simulink model "RealtimeModel"  (Simulink 7.0)
settings: Solver=FixedStepDiscrete  SolverMode=MultiTasking  StartTime=0.0  StopTime=RunningTime  FixedStep=sample  RelTol=1e-3
values from neighbouring files (symbols this model uses):
  Integrator = InitializeIntegrator(Integrator, Structure)    [RealtimeModel_Setup.m]
  Interpolations = SampleRate/sample    [RealtimeModel_Setup.m]
  sample = 1/1024    (= 0.0009765625)    [RealtimeModel_Setup.m]
  SampleRate = Integrator.Timestep    [RealtimeModel_Setup.m]
undefined symbols (not defined in the file or in its folder): Elements
(part 3 of 3)

== matlab function Generate Element Restoring Forces/Generate Type 3 Element Restoring Force Element 2/Type 3 Element RF ==
  data: TotalRF output inherited; Element input inherited; a1 input inherited; a2 input inherited; pmx input inherited; bmy_init input inherited; Displacement input inherited; NumFreeDOF parameter inherited
% Get Restoring Force Type 3
function TotalRF  = fnc(Element, a1, a2, pmx, bmy_init, Displacement, NumFreeDOF)

persistent initialized;
persistent kody;
persistent bmep;
persistent bmel;
persistent bmtot;
persistent bbmy;
persistent dpr;
persistent bmy;
persistent ftot;
persistent pracn;
persistent pracp;
persistent prtot;
persistent sftot;
persistent Uprev;

%% Input mapping
ksurf = Element(1);
cosa = Element(2);
eal = Element(3);
ek11 = Element(4);
ek11h = Element(5);
ek12 = Element(6);
ek22 = Element(7);
ek22h = Element(8);
fl = Element(9);
pr12 = Element(10);
pr21 = Element(11);
psh = Element(12);
sina = Element(13);
Node1UX = Element(14);
Node1UY = Element(15);
Node1THETA = Element(16);
Node2UX = Element(17);
Node2UY = Element(18);
Node2THETA = Element(19);

if isempty(initialized)
    initialized = 1;
    kody = zeros(2,1);
    bmep = zeros(2,1); 
    bmel = zeros(2,1);
    bmtot = zeros(2,1);
    bbmy = 0;
    dpr = zeros(2,1);
    ftot = zeros(2,1);  
    pracn = zeros(2,1); 
    pracp = zeros(2,1);
    prtot = zeros(2,1);
    sftot = zeros(2,1); 
    Uprev = zeros(6,1);
    bmy = bmy_init;
end

%% Get the displacement Ue (6x1) vector of the element in global coordinates
Ue = zeros(6,1);
dof=zeros(6,1);
dof(1,1)=Node1UX;
dof(2,1)=Node1UY;
dof(3,1)=Node1THETA;
dof(4,1)=Node2UX;
dof(5,1)=Node2UY;
dof(6,1)=Node2THETA;
for i=1:6
    if dof(i,1)<=NumFreeDOF
        Ue(i,1)=Displacement(dof(i,1),1);
    end
end

%% Input of Drain State Determination Type 2 Element
ndof=6;  %the element has 6 dofs
ddise=Ue-Uprev;  %the incremental displacement vector ddise of the element in global coordinates 
Uprev=Ue; %update Uprev of element for use in next state determination call
%% calculate element deformation increments
[dvax,dvr] = ELDFO2(ddise,fl,cosa,sina);
%% UPDATE AXIAL FORCES AND AXIAL ENERGY
dfax=eal*dvax;      
ftot(1,1)=ftot(1,1)-dfax;
ftot(2,1)=ftot(2,1)+dfax;  
%% MOMENTS IN ELASTIC COMPONENT AT BEGINING OF STEP
bmel(1,1)=bmtot(1,1)-bmep(1,1);
bmel(2,1)=bmtot(2,1)-bmep(2,1);
%% LINEAR MOMENT INCREMENTS FOR ELASTO-PLASTIC COMPONENT - SET IN DBM
[dbm] = BMCAO2(dvr,kody,ek11,ek12,ek22,ek22h,ek11h);
%% TRACE NONLINEAR PATH FOR ELASTO-PLASTIC COMPONENT---state determination
facac=0.0;
while (facac<0.999999)
    factor=1.0-facac;
    % PLASTIC HINGE ROTATIONS
    kod=kody(1,1)+kody(2,1)-1.0;
    if(kod>0)
        % hinges at both ends
        dpr(1,1)=dvr(1,1);
        dpr(2,1)=dvr(2,1);
    elseif(kod==0)
        % hinge at one end only
        dpr(1,1)=dvr(1,1)+pr21*dvr(2,1);
        dpr(2,1)=dvr(2,1)+pr12*dvr(1,1);
    else
         %never executed
    end
         
    % CALCULATE WHICH END HAS NEXT EVENT IF YIELDS, SET KFAC=IEND AND BBMY=YIELD VALUE
    % SET EVENT FACTOR IN FACTOR
    kfac=3;
    for iend=1:2
        if (kody(iend,1)==0.0)
            dbmm=dbm(iend,1);
            % elastic, get factor for status change(no hinge at end)
            if (dbmm<0.0)
                dbmo=bmy(iend,2)-bmep(iend,1);
                if(dbmo>=dbmm) 
                    fac=dbmo/dbmm;
                else
                    fac=2.0;
                end 
                if (fac<=factor)
                    factor=fac;
                    bbmy=bmy(iend,2);
                    kfac=iend;
                end
            elseif(dbmm>0.0)
                dbmo=bmy(iend,1)-bmep(iend,1);
                if(dbmo<=dbmm) 
                    fac=dbmo/dbmm;
                else
                    fac=2.0;
                end 
                if (fac<=factor)
                    factor=fac;
                    bbmy=bmy(iend,1);
                    kfac=iend;
                end
            else
            end
        else
            % hinge at this end
            if(bmep(iend,1)*dpr(iend,1)<0.0)
            % unloading (plastic work negative)
                factor=0.0;
                kfac=0.0;
                kody(iend,1)=0.0;
            else
                % continuing to yield (plastic work positive)
            end
        end
    end
    % UPDATE BENDING STATE AND CALCULATE BENDING ENERGY
    % dbm= elastic increment - use if elastic bbmy= yield value - use if yields
    if(kfac~=0)
        for iend=1:2
            if(iend==kfac)
                % new hinge at this end
                bmep(iend,1)=bbmy;
                kody(iend,1)=1;
            elseif(kody(iend,1)==0)
                % this end remains elastic
                dmep=factor*dbm(iend,1);
                bmep(iend,1)=bmep(iend,1)+dmep;
            else
                % this end remains plastic
                dppr=factor*dpr(iend,1);
                prtot(iend,1)=prtot(iend,1)+dppr;
                if (dppr<0.0)
                    pracn(iend,1)=pracn(iend,1)+dppr;
                else
                    pracp(iend,1)=pracp(iend,1)+dppr;
                end
            end
        end
    else
        % unloads - factor=0.
    end
    % CHECK COMPLETION OF CYCLE
    facac=facac+factor;
    if (facac<0.99999)
        % cycle not completed, calculate new moment increments
        [dbm] = BMCAO2(dvr,kody,ek11,ek12,ek22,ek22h,ek11h);
    end
end
%% YIELD MOMENTS FOR NEXT STEP
if(ksurf==1)
    [bmy] = YMOM02(ftot,pmx,a1,a2,bmy);
    % CHECK YIELD SURFACE OVERSHOOT
    for iend=1:2
        if (kody(iend,1)~=0.0)
        % inelastic on old surface
            if (bmep(iend,1)>bmy(iend,1)) 
                % inelastic positive on new surface also
                bmep(iend,1)=bmy(iend,1);
            elseif (bmep(iend,1)<bmy(iend,2))
                % inelastic negative on new surface also
                bmep(iend,1)=bmy(iend,2);
            elseif ((bmep(iend,1)<(bmy(iend,1)*0.98)) && (bmep(iend,1)>(bmy(iend,2)*0.98)))
                % moves inside new surface by > 2% - reset yield code
                kody(iend,1)=0;
            else
            end
        else
            % elastic on old surface
            if (bmep(iend,1)>bmy(iend,1))
                % inelastic positive on new surface
                bmep(iend,1)=bmy(iend,1);
                kody(iend,1)=1;
            elseif (bmep(iend,1)<=bmy(iend,2))
                % inelastic negative on new surface
                bmep(iend,1)=bmy(iend,2);
                kody(iend,1)=1;
            else
            end
        end
    end
end
%% UPDATE TOTAL FORCES
dsf=(bmtot(1,1)+ bmtot(2,1))/fl;
ppsh=psh/(1.0-psh);
dmeli=(ek11*dvr(1,1)+ek12*dvr(2,1))*ppsh+bmel(1,1);
dmelj=(ek12*dvr(1,1)+ ek22*dvr(2,1))*ppsh+bmel(2,1);
bmtot(1,1)=bmep(1,1)+dmeli;
bmtot(2,1)=bmep(2,1)+dmelj;
dsf=dsf-(bmtot(1,1)+bmtot(2,1))/fl;
sftot(1,1)=sftot(1,1)-dsf;
sftot(2,1)=sftot(2,1)+dsf;

RF = ELASO2(ndof,ftot,cosa,sina,sftot,bmtot);

% Form total restoring force vector
TotalRF = zeros(NumFreeDOF, 1);
    
% Get element nodes to assemble in the structure restoring force vector
if Node1UX <= NumFreeDOF
    TotalRF(Node1UX, 1) = RF(1, 1);
end
if Node1UY <= NumFreeDOF
    TotalRF(Node1UY, 1) = RF(2, 1);
end
if Node1THETA <= NumFreeDOF
    TotalRF(Node1THETA, 1) = RF(3, 1);
end
if Node2UX <= NumFreeDOF
    TotalRF(Node2UX, 1) = RF(4, 1);
end
if Node2UY <= NumFreeDOF
    TotalRF(Node2UY, 1) = RF(5, 1);
end
if Node2THETA <= NumFreeDOF
    TotalRF(Node2THETA, 1) = RF(6, 1);
end





%%%%%%% FUNCTIONS %%%%%%%%%
function [bmy] = YMOM02(ftot,pmx,a1,a2,bmy)
facc=-1.0;
for iend = 1 : 2
    % Change sign of axial force and end 1
    fft = ftot(iend,1) * facc;
    facc = 1;
    fac = 1;
    for j = 1 : 2
        fac = -fac;
        yieldcalc = 0;  % flag if the yield moment is calculated inside 
                        % this next for loop
        for i = 1 : 3
            if (fft < pmx(i,j,iend))
                yieldcalc = 1;  % set flag since the condition was met
                % Calculate yield moment (M = a2 + a1P)
                bbmy = a2(i,j,iend) - a1(i,j,iend) * fft;
                if (fac * bbmy > 0) 
                    % Axial force is beyond Pc and Pt
                    bbmy = 0;
                end
                bmy(iend,j) = bbmy;
            end
        end
        % Only calculate yield moment if it wasn't calculated in the above
        % for loop
        if (yieldcalc == 0)
            i = 4;
            % Calculate yield moment (M = a2 + a1P)
            bbmy = a2(i,j,iend) - a1(i,j,iend) * fft;
            if (fac * bbmy > 0) 
                % Axial force is beyond Pc and Pt
                bbmy = 0;
            end
            bmy(iend,j) = bbmy;
        end
    end
end
%c ---------------------------------INTERCHANGE BMY(1,1) AND BMY(1,2) AND
%c ------------------------------AND ALSO CHANGE SIGN OF MOMENTS AT END 1
fac=-bmy(1,1);
bmy(1,1)=-bmy(1,2);
bmy(1,2)=fac;
      
      
      
      
      
function [dbm] = BMCAO2(dvr,kody,ek11,ek12,ek22,ek22h,ek11h)
dbm=zeros(2,1);
% c ------------------SET KYY TO INDICATE TYPE OF ELEMENT STIFFNESS TO USE
      kyy=kody(1,1)+2*kody(2,1)+1;
      if(kyy==1)
%c---no hinge at either end
        dbm(1,1)=ek11*dvr(1,1)+ek12*dvr(2,1);
        dbm(2,1)=ek12*dvr(1,1)+ek22*dvr(2,1);
      elseif(kyy==2)
%c---hinge at end 1
        dbm(1,1)=0.0;
        dbm(2,1)=ek22h*dvr(2,1);
      elseif(kyy==3)
%c---hinge at end 2
        dbm(1,1)=ek11h*dvr(1,1);
        dbm(2,1)=0.0;
      elseif(kyy==4)
%c---hinges at both end
        dbm(1,1)=0.0;
        dbm(2,1)=0.0;
       else
           %never executed
      end
      
      
      
      
      
      
      
      
      
      
   %%
function [relas] = ELASO2(ndof,ftot,cosa,sina,sftot,bmtot)
%%
relas=zeros(ndof,1);
%BASIC RESISTING FORCES
      relas(1,1)=(ftot(1,1)-0)*cosa-(sftot(1,1)-0)*sina;
      relas(2,1)=(ftot(1,1)-0)*sina+(sftot(1,1)-0)*cosa;
      relas(3,1)=bmtot(1,1)-0-0;
      relas(4,1)=(ftot(2,1)-0)*cosa-(sftot(2,1)-0)*sina;
      relas(5,1)=(ftot(2,1)-0)*sina+(sftot(2,1)-0)*cosa;
      relas(6,1)=bmtot(2,1)-0-0;
%%







%%
function [dvax,dvr] = ELDFO2(ddise,f1,cosa, sina) 
%%
dvr=zeros(2,1);
%DEFORMATION INCREMENTS OR DEFORMATION RATES
      dvax=cosa*(ddise(4,1)-ddise(1,1))+sina*(ddise(5,1)-ddise(2,1));
      rot=(sina*(ddise(4,1)-ddise(1,1))+cosa*(ddise(2,1)-ddise(5,1)))/f1;
      dvr(1,1)=ddise(3,1)+rot;
      dvr(2,1)=ddise(6,1)+rot;
%%

== matlab function Generate Element Restoring Forces/Generate Type 3 Element Restoring Force Element 4/Type 3 Element RF ==
  data: TotalRF output inherited; Element input inherited; a1 input inherited; a2 input inherited; pmx input inherited; bmy_init input inherited; Displacement input inherited; NumFreeDOF parameter inherited
% Get Restoring Force Type 3
function TotalRF  = fnc(Element, a1, a2, pmx, bmy_init, Displacement, NumFreeDOF)

persistent initialized;
persistent kody;
persistent bmep;
persistent bmel;
persistent bmtot;
persistent bbmy;
persistent dpr;
persistent bmy;
persistent ftot;
persistent pracn;
persistent pracp;
persistent prtot;
persistent sftot;
persistent Uprev;

%% Input mapping
ksurf = Element(1);
cosa = Element(2);
eal = Element(3);
ek11 = Element(4);
ek11h = Element(5);
ek12 = Element(6);
ek22 = Element(7);
ek22h = Element(8);
fl = Element(9);
pr12 = Element(10);
pr21 = Element(11);
psh = Element(12);
sina = Element(13);
Node1UX = Element(14);
Node1UY = Element(15);
Node1THETA = Element(16);
Node2UX = Element(17);
Node2UY = Element(18);
Node2THETA = Element(19);

if isempty(initialized)
    initialized = 1;
    kody = zeros(2,1);
    bmep = zeros(2,1); 
    bmel = zeros(2,1);
    bmtot = zeros(2,1);
    bbmy = 0;
    dpr = zeros(2,1);
    ftot = zeros(2,1);  
    pracn = zeros(2,1); 
    pracp = zeros(2,1);
    prtot = zeros(2,1);
    sftot = zeros(2,1); 
    Uprev = zeros(6,1);
    bmy = bmy_init;
end

%% Get the displacement Ue (6x1) vector of the element in global coordinates
Ue = zeros(6,1);
dof=zeros(6,1);
dof(1,1)=Node1UX;
dof(2,1)=Node1UY;
dof(3,1)=Node1THETA;
dof(4,1)=Node2UX;
dof(5,1)=Node2UY;
dof(6,1)=Node2THETA;
for i=1:6
    if dof(i,1)<=NumFreeDOF
        Ue(i,1)=Displacement(dof(i,1),1);
    end
end

%% Input of Drain State Determination Type 2 Element
ndof=6;  %the element has 6 dofs
ddise=Ue-Uprev;  %the incremental displacement vector ddise of the element in global coordinates 
Uprev=Ue; %update Uprev of element for use in next state determination call
%% calculate element deformation increments
[dvax,dvr] = ELDFO2(ddise,fl,cosa,sina);
%% UPDATE AXIAL FORCES AND AXIAL ENERGY
dfax=eal*dvax;      
ftot(1,1)=ftot(1,1)-dfax;
ftot(2,1)=ftot(2,1)+dfax;  
%% MOMENTS IN ELASTIC COMPONENT AT BEGINING OF STEP
bmel(1,1)=bmtot(1,1)-bmep(1,1);
bmel(2,1)=bmtot(2,1)-bmep(2,1);
%% LINEAR MOMENT INCREMENTS FOR ELASTO-PLASTIC COMPONENT - SET IN DBM
[dbm] = BMCAO2(dvr,kody,ek11,ek12,ek22,ek22h,ek11h);
%% TRACE NONLINEAR PATH FOR ELASTO-PLASTIC COMPONENT---state determination
facac=0.0;
while (facac<0.999999)
    factor=1.0-facac;
    % PLASTIC HINGE ROTATIONS
    kod=kody(1,1)+kody(2,1)-1.0;
    if(kod>0)
        % hinges at both ends
        dpr(1,1)=dvr(1,1);
        dpr(2,1)=dvr(2,1);
    elseif(kod==0)
        % hinge at one end only
        dpr(1,1)=dvr(1,1)+pr21*dvr(2,1);
        dpr(2,1)=dvr(2,1)+pr12*dvr(1,1);
    else
         %never executed
    end
         
    % CALCULATE WHICH END HAS NEXT EVENT IF YIELDS, SET KFAC=IEND AND BBMY=YIELD VALUE
    % SET EVENT FACTOR IN FACTOR
    kfac=3;
    for iend=1:2
        if (kody(iend,1)==0.0)
            dbmm=dbm(iend,1);
            % elastic, get factor for status change(no hinge at end)
            if (dbmm<0.0)
                dbmo=bmy(iend,2)-bmep(iend,1);
                if(dbmo>=dbmm) 
                    fac=dbmo/dbmm;
                else
                    fac=2.0;
                end 
                if (fac<=factor)
                    factor=fac;
                    bbmy=bmy(iend,2);
                    kfac=iend;
                end
            elseif(dbmm>0.0)
                dbmo=bmy(iend,1)-bmep(iend,1);
                if(dbmo<=dbmm) 
                    fac=dbmo/dbmm;
                else
                    fac=2.0;
                end 
                if (fac<=factor)
                    factor=fac;
                    bbmy=bmy(iend,1);
                    kfac=iend;
                end
            else
            end
        else
            % hinge at this end
            if(bmep(iend,1)*dpr(iend,1)<0.0)
            % unloading (plastic work negative)
                factor=0.0;
                kfac=0.0;
                kody(iend,1)=0.0;
            else
                % continuing to yield (plastic work positive)
            end
        end
    end
    % UPDATE BENDING STATE AND CALCULATE BENDING ENERGY
    % dbm= elastic increment - use if elastic bbmy= yield value - use if yields
    if(kfac~=0)
        for iend=1:2
            if(iend==kfac)
                % new hinge at this end
                bmep(iend,1)=bbmy;
                kody(iend,1)=1;
            elseif(kody(iend,1)==0)
                % this end remains elastic
                dmep=factor*dbm(iend,1);
                bmep(iend,1)=bmep(iend,1)+dmep;
            else
                % this end remains plastic
                dppr=factor*dpr(iend,1);
                prtot(iend,1)=prtot(iend,1)+dppr;
                if (dppr<0.0)
                    pracn(iend,1)=pracn(iend,1)+dppr;
                else
                    pracp(iend,1)=pracp(iend,1)+dppr;
                end
            end
        end
    else
        % unloads - factor=0.
    end
    % CHECK COMPLETION OF CYCLE
    facac=facac+factor;
    if (facac<0.99999)
        % cycle not completed, calculate new moment increments
        [dbm] = BMCAO2(dvr,kody,ek11,ek12,ek22,ek22h,ek11h);
    end
end
%% YIELD MOMENTS FOR NEXT STEP
if(ksurf==1)
    [bmy] = YMOM02(ftot,pmx,a1,a2,bmy);
    % CHECK YIELD SURFACE OVERSHOOT
    for iend=1:2
        if (kody(iend,1)~=0.0)
        % inelastic on old surface
            if (bmep(iend,1)>bmy(iend,1)) 
                % inelastic positive on new surface also
                bmep(iend,1)=bmy(iend,1);
            elseif (bmep(iend,1)<bmy(iend,2))
                % inelastic negative on new surface also
                bmep(iend,1)=bmy(iend,2);
            elseif ((bmep(iend,1)<(bmy(iend,1)*0.98)) && (bmep(iend,1)>(bmy(iend,2)*0.98)))
                % moves inside new surface by > 2% - reset yield code
                kody(iend,1)=0;
            else
            end
        else
            % elastic on old surface
            if (bmep(iend,1)>bmy(iend,1))
                % inelastic positive on new surface
                bmep(iend,1)=bmy(iend,1);
                kody(iend,1)=1;
            elseif (bmep(iend,1)<=bmy(iend,2))
                % inelastic negative on new surface
                bmep(iend,1)=bmy(iend,2);
                kody(iend,1)=1;
            else
            end
        end
    end
end
%% UPDATE TOTAL FORCES
dsf=(bmtot(1,1)+ bmtot(2,1))/fl;
ppsh=psh/(1.0-psh);
dmeli=(ek11*dvr(1,1)+ek12*dvr(2,1))*ppsh+bmel(1,1);
dmelj=(ek12*dvr(1,1)+ ek22*dvr(2,1))*ppsh+bmel(2,1);
bmtot(1,1)=bmep(1,1)+dmeli;
bmtot(2,1)=bmep(2,1)+dmelj;
dsf=dsf-(bmtot(1,1)+bmtot(2,1))/fl;
sftot(1,1)=sftot(1,1)-dsf;
sftot(2,1)=sftot(2,1)+dsf;

RF = ELASO2(ndof,ftot,cosa,sina,sftot,bmtot);

% Form total restoring force vector
TotalRF = zeros(NumFreeDOF, 1);
    
% Get element nodes to assemble in the structure restoring force vector
if Node1UX <= NumFreeDOF
    TotalRF(Node1UX, 1) = RF(1, 1);
end
if Node1UY <= NumFreeDOF
    TotalRF(Node1UY, 1) = RF(2, 1);
end
if Node1THETA <= NumFreeDOF
    TotalRF(Node1THETA, 1) = RF(3, 1);
end
if Node2UX <= NumFreeDOF
    TotalRF(Node2UX, 1) = RF(4, 1);
end
if Node2UY <= NumFreeDOF
    TotalRF(Node2UY, 1) = RF(5, 1);
end
if Node2THETA <= NumFreeDOF
    TotalRF(Node2THETA, 1) = RF(6, 1);
end





%%%%%%% FUNCTIONS %%%%%%%%%
function [bmy] = YMOM02(ftot,pmx,a1,a2,bmy)
facc=-1.0;
for iend = 1 : 2
    % Change sign of axial force and end 1
    fft = ftot(iend,1) * facc;
    facc = 1;
    fac = 1;
    for j = 1 : 2
        fac = -fac;
        yieldcalc = 0;  % flag if the yield moment is calculated inside 
                        % this next for loop
        for i = 1 : 3
            if (fft < pmx(i,j,iend))
                yieldcalc = 1;  % set flag since the condition was met
                % Calculate yield moment (M = a2 + a1P)
                bbmy = a2(i,j,iend) - a1(i,j,iend) * fft;
                if (fac * bbmy > 0) 
                    % Axial force is beyond Pc and Pt
                    bbmy = 0;
                end
                bmy(iend,j) = bbmy;
            end
        end
        % Only calculate yield moment if it wasn't calculated in the above
        % for loop
        if (yieldcalc == 0)
            i = 4;
            % Calculate yield moment (M = a2 + a1P)
            bbmy = a2(i,j,iend) - a1(i,j,iend) * fft;
            if (fac * bbmy > 0) 
                % Axial force is beyond Pc and Pt
                bbmy = 0;
            end
            bmy(iend,j) = bbmy;
        end
    end
end
%c ---------------------------------INTERCHANGE BMY(1,1) AND BMY(1,2) AND
%c ------------------------------AND ALSO CHANGE SIGN OF MOMENTS AT END 1
fac=-bmy(1,1);
bmy(1,1)=-bmy(1,2);
bmy(1,2)=fac;
      
      
      
      
      
function [dbm] = BMCAO2(dvr,kody,ek11,ek12,ek22,ek22h,ek11h)
dbm=zeros(2,1);
% c ------------------SET KYY TO INDICATE TYPE OF ELEMENT STIFFNESS TO USE
      kyy=kody(1,1)+2*kody(2,1)+1;
      if(kyy==1)
%c---no hinge at either end
        dbm(1,1)=ek11*dvr(1,1)+ek12*dvr(2,1);
        dbm(2,1)=ek12*dvr(1,1)+ek22*dvr(2,1);
      elseif(kyy==2)
%c---hinge at end 1
        dbm(1,1)=0.0;
        dbm(2,1)=ek22h*dvr(2,1);
      elseif(kyy==3)
%c---hinge at end 2
        dbm(1,1)=ek11h*dvr(1,1);
        dbm(2,1)=0.0;
      elseif(kyy==4)
%c---hinges at both end
        dbm(1,1)=0.0;
        dbm(2,1)=0.0;
       else
           %never executed
      end
      
      
      
      
      
      
      
      
      
      
   %%
function [relas] = ELASO2(ndof,ftot,cosa,sina,sftot,bmtot)
%%
relas=zeros(ndof,1);
%BASIC RESISTING FORCES
      relas(1,1)=(ftot(1,1)-0)*cosa-(sftot(1,1)-0)*sina;
      relas(2,1)=(ftot(1,1)-0)*sina+(sftot(1,1)-0)*cosa;
      relas(3,1)=bmtot(1,1)-0-0;
      relas(4,1)=(ftot(2,1)-0)*cosa-(sftot(2,1)-0)*sina;
      relas(5,1)=(ftot(2,1)-0)*sina+(sftot(2,1)-0)*cosa;
      relas(6,1)=bmtot(2,1)-0-0;
%%







%%
function [dvax,dvr] = ELDFO2(ddise,f1,cosa, sina) 
%%
dvr=zeros(2,1);
%DEFORMATION INCREMENTS OR DEFORMATION RATES
      dvax=cosa*(ddise(4,1)-ddise(1,1))+sina*(ddise(5,1)-ddise(2,1));
      rot=(sina*(ddise(4,1)-ddise(1,1))+cosa*(ddise(2,1)-ddise(5,1)))/f1;
      dvr(1,1)=ddise(3,1)+rot;
      dvr(2,1)=ddise(6,1)+rot;
%%

== matlab function Generate Element Restoring Forces/Generate Type 3 Element Restoring Force Element 5/Type 3 Element RF ==
  data: TotalRF output inherited; Element input inherited; a1 input inherited; a2 input inherited; pmx input inherited; bmy_init input inherited; Displacement input inherited; NumFreeDOF parameter inherited
% Get Restoring Force Type 3
function TotalRF  = fnc(Element, a1, a2, pmx, bmy_init, Displacement, NumFreeDOF)

persistent initialized;
persistent kody;
persistent bmep;
persistent bmel;
persistent bmtot;
persistent bbmy;
persistent dpr;
persistent bmy;
persistent ftot;
persistent pracn;
persistent pracp;
persistent prtot;
persistent sftot;
persistent Uprev;

%% Input mapping
ksurf = Element(1);
cosa = Element(2);
eal = Element(3);
ek11 = Element(4);
ek11h = Element(5);
ek12 = Element(6);
ek22 = Element(7);
ek22h = Element(8);
fl = Element(9);
pr12 = Element(10);
pr21 = Element(11);
psh = Element(12);
sina = Element(13);
Node1UX = Element(14);
Node1UY = Element(15);
Node1THETA = Element(16);
Node2UX = Element(17);
Node2UY = Element(18);
Node2THETA = Element(19);

if isempty(initialized)
    initialized = 1;
    kody = zeros(2,1);
    bmep = zeros(2,1); 
    bmel = zeros(2,1);
    bmtot = zeros(2,1);
    bbmy = 0;
    dpr = zeros(2,1);
    ftot = zeros(2,1);  
    pracn = zeros(2,1); 
    pracp = zeros(2,1);
    prtot = zeros(2,1);
    sftot = zeros(2,1); 
    Uprev = zeros(6,1);
    bmy = bmy_init;
end

%% Get the displacement Ue (6x1) vector of the element in global coordinates
Ue = zeros(6,1);
dof=zeros(6,1);
dof(1,1)=Node1UX;
dof(2,1)=Node1UY;
dof(3,1)=Node1THETA;
dof(4,1)=Node2UX;
dof(5,1)=Node2UY;
dof(6,1)=Node2THETA;
for i=1:6
    if dof(i,1)<=NumFreeDOF
        Ue(i,1)=Displacement(dof(i,1),1);
    end
end

%% Input of Drain State Determination Type 2 Element
ndof=6;  %the element has 6 dofs
ddise=Ue-Uprev;  %the incremental displacement vector ddise of the element in global coordinates 
Uprev=Ue; %update Uprev of element for use in next state determination call
%% calculate element deformation increments
[dvax,dvr] = ELDFO2(ddise,fl,cosa,sina);
%% UPDATE AXIAL FORCES AND AXIAL ENERGY
dfax=eal*dvax;      
ftot(1,1)=ftot(1,1)-dfax;
ftot(2,1)=ftot(2,1)+dfax;  
%% MOMENTS IN ELASTIC COMPONENT AT BEGINING OF STEP
bmel(1,1)=bmtot(1,1)-bmep(1,1);
bmel(2,1)=bmtot(2,1)-bmep(2,1);
%% LINEAR MOMENT INCREMENTS FOR ELASTO-PLASTIC COMPONENT - SET IN DBM
[dbm] = BMCAO2(dvr,kody,ek11,ek12,ek22,ek22h,ek11h);
%% TRACE NONLINEAR PATH FOR ELASTO-PLASTIC COMPONENT---state determination
facac=0.0;
while (facac<0.999999)
    factor=1.0-facac;
    % PLASTIC HINGE ROTATIONS
    kod=kody(1,1)+kody(2,1)-1.0;
    if(kod>0)
        % hinges at both ends
        dpr(1,1)=dvr(1,1);
        dpr(2,1)=dvr(2,1);
    elseif(kod==0)
        % hinge at one end only
        dpr(1,1)=dvr(1,1)+pr21*dvr(2,1);
        dpr(2,1)=dvr(2,1)+pr12*dvr(1,1);
    else
         %never executed
    end
         
    % CALCULATE WHICH END HAS NEXT EVENT IF YIELDS, SET KFAC=IEND AND BBMY=YIELD VALUE
    % SET EVENT FACTOR IN FACTOR
    kfac=3;
    for iend=1:2
        if (kody(iend,1)==0.0)
            dbmm=dbm(iend,1);
            % elastic, get factor for status change(no hinge at end)
            if (dbmm<0.0)
                dbmo=bmy(iend,2)-bmep(iend,1);
                if(dbmo>=dbmm) 
                    fac=dbmo/dbmm;
                else
                    fac=2.0;
                end 
                if (fac<=factor)
                    factor=fac;
                    bbmy=bmy(iend,2);
                    kfac=iend;
                end
            elseif(dbmm>0.0)
                dbmo=bmy(iend,1)-bmep(iend,1);
                if(dbmo<=dbmm) 
                    fac=dbmo/dbmm;
                else
                    fac=2.0;
                end 
                if (fac<=factor)
                    factor=fac;
                    bbmy=bmy(iend,1);
                    kfac=iend;
                end
            else
            end
        else
            % hinge at this end
            if(bmep(iend,1)*dpr(iend,1)<0.0)
            % unloading (plastic work negative)
                factor=0.0;
                kfac=0.0;
                kody(iend,1)=0.0;
            else
                % continuing to yield (plastic work positive)
            end
        end
    end
    % UPDATE BENDING STATE AND CALCULATE BENDING ENERGY
    % dbm= elastic increment - use if elastic bbmy= yield value - use if yields
    if(kfac~=0)
        for iend=1:2
            if(iend==kfac)
                % new hinge at this end
                bmep(iend,1)=bbmy;
                kody(iend,1)=1;
            elseif(kody(iend,1)==0)
                % this end remains elastic
                dmep=factor*dbm(iend,1);
                bmep(iend,1)=bmep(iend,1)+dmep;
            else
                % this end remains plastic
                dppr=factor*dpr(iend,1);
                prtot(iend,1)=prtot(iend,1)+dppr;
                if (dppr<0.0)
                    pracn(iend,1)=pracn(iend,1)+dppr;
                else
                    pracp(iend,1)=pracp(iend,1)+dppr;
                end
            end
        end
    else
        % unloads - factor=0.
    end
    % CHECK COMPLETION OF CYCLE
    facac=facac+factor;
    if (facac<0.99999)
        % cycle not completed, calculate new moment increments
        [dbm] = BMCAO2(dvr,kody,ek11,ek12,ek22,ek22h,ek11h);
    end
end
%% YIELD MOMENTS FOR NEXT STEP
if(ksurf==1)
    [bmy] = YMOM02(ftot,pmx,a1,a2,bmy);
    % CHECK YIELD SURFACE OVERSHOOT
    for iend=1:2
        if (kody(iend,1)~=0.0)
        % inelastic on old surface
            if (bmep(iend,1)>bmy(iend,1)) 
                % inelastic positive on new surface also
                bmep(iend,1)=bmy(iend,1);
            elseif (bmep(iend,1)<bmy(iend,2))
                % inelastic negative on new surface also
                bmep(iend,1)=bmy(iend,2);
            elseif ((bmep(iend,1)<(bmy(iend,1)*0.98)) && (bmep(iend,1)>(bmy(iend,2)*0.98)))
                % moves inside new surface by > 2% - reset yield code
                kody(iend,1)=0;
            else
            end
        else
            % elastic on old surface
            if (bmep(iend,1)>bmy(iend,1))
                % inelastic positive on new surface
                bmep(iend,1)=bmy(iend,1);
                kody(iend,1)=1;
            elseif (bmep(iend,1)<=bmy(iend,2))
                % inelastic negative on new surface
                bmep(iend,1)=bmy(iend,2);
                kody(iend,1)=1;
            else
            end
        end
    end
end
%% UPDATE TOTAL FORCES
dsf=(bmtot(1,1)+ bmtot(2,1))/fl;
ppsh=psh/(1.0-psh);
dmeli=(ek11*dvr(1,1)+ek12*dvr(2,1))*ppsh+bmel(1,1);
dmelj=(ek12*dvr(1,1)+ ek22*dvr(2,1))*ppsh+bmel(2,1);
bmtot(1,1)=bmep(1,1)+dmeli;
bmtot(2,1)=bmep(2,1)+dmelj;
dsf=dsf-(bmtot(1,1)+bmtot(2,1))/fl;
sftot(1,1)=sftot(1,1)-dsf;
sftot(2,1)=sftot(2,1)+dsf;

RF = ELASO2(ndof,ftot,cosa,sina,sftot,bmtot);

% Form total restoring force vector
TotalRF = zeros(NumFreeDOF, 1);
    
% Get element nodes to assemble in the structure restoring force vector
if Node1UX <= NumFreeDOF
    TotalRF(Node1UX, 1) = RF(1, 1);
end
if Node1UY <= NumFreeDOF
    TotalRF(Node1UY, 1) = RF(2, 1);
end
if Node1THETA <= NumFreeDOF
    TotalRF(Node1THETA, 1) = RF(3, 1);
end
if Node2UX <= NumFreeDOF
    TotalRF(Node2UX, 1) = RF(4, 1);
end
if Node2UY <= NumFreeDOF
    TotalRF(Node2UY, 1) = RF(5, 1);
end
if Node2THETA <= NumFreeDOF
    TotalRF(Node2THETA, 1) = RF(6, 1);
end





%%%%%%% FUNCTIONS %%%%%%%%%
function [bmy] = YMOM02(ftot,pmx,a1,a2,bmy)
facc=-1.0;
for iend = 1 : 2
    % Change sign of axial force and end 1
    fft = ftot(iend,1) * facc;
    facc = 1;
    fac = 1;
    for j = 1 : 2
        fac = -fac;
        yieldcalc = 0;  % flag if the yield moment is calculated inside 
                        % this next for loop
        for i = 1 : 3
            if (fft < pmx(i,j,iend))
                yieldcalc = 1;  % set flag since the condition was met
                % Calculate yield moment (M = a2 + a1P)
                bbmy = a2(i,j,iend) - a1(i,j,iend) * fft;
                if (fac * bbmy > 0) 
                    % Axial force is beyond Pc and Pt
                    bbmy = 0;
                end
                bmy(iend,j) = bbmy;
            end
        end
        % Only calculate yield moment if it wasn't calculated in the above
        % for loop
        if (yieldcalc == 0)
            i = 4;
            % Calculate yield moment (M = a2 + a1P)
            bbmy = a2(i,j,iend) - a1(i,j,iend) * fft;
            if (fac * bbmy > 0) 
                % Axial force is beyond Pc and Pt
                bbmy = 0;
            end
            bmy(iend,j) = bbmy;
        end
    end
end
%c ---------------------------------INTERCHANGE BMY(1,1) AND BMY(1,2) AND
%c ------------------------------AND ALSO CHANGE SIGN OF MOMENTS AT END 1
fac=-bmy(1,1);
bmy(1,1)=-bmy(1,2);
bmy(1,2)=fac;
      
      
      
      
      
function [dbm] = BMCAO2(dvr,kody,ek11,ek12,ek22,ek22h,ek11h)
dbm=zeros(2,1);
% c ------------------SET KYY TO INDICATE TYPE OF ELEMENT STIFFNESS TO USE
      kyy=kody(1,1)+2*kody(2,1)+1;
      if(kyy==1)
%c---no hinge at either end
        dbm(1,1)=ek11*dvr(1,1)+ek12*dvr(2,1);
        dbm(2,1)=ek12*dvr(1,1)+ek22*dvr(2,1);
      elseif(kyy==2)
%c---hinge at end 1
        dbm(1,1)=0.0;
        dbm(2,1)=ek22h*dvr(2,1);
      elseif(kyy==3)
%c---hinge at end 2
        dbm(1,1)=ek11h*dvr(1,1);
        dbm(2,1)=0.0;
      elseif(kyy==4)
%c---hinges at both end
        dbm(1,1)=0.0;
        dbm(2,1)=0.0;
       else
           %never executed
      end
      
      
      
      
      
      
      
      
      
      
   %%
function [relas] = ELASO2(ndof,ftot,cosa,sina,sftot,bmtot)
%%
relas=zeros(ndof,1);
%BASIC RESISTING FORCES
      relas(1,1)=(ftot(1,1)-0)*cosa-(sftot(1,1)-0)*sina;
      relas(2,1)=(ftot(1,1)-0)*sina+(sftot(1,1)-0)*cosa;
      relas(3,1)=bmtot(1,1)-0-0;
      relas(4,1)=(ftot(2,1)-0)*cosa-(sftot(2,1)-0)*sina;
      relas(5,1)=(ftot(2,1)-0)*sina+(sftot(2,1)-0)*cosa;
      relas(6,1)=bmtot(2,1)-0-0;
%%







%%
function [dvax,dvr] = ELDFO2(ddise,f1,cosa, sina) 
%%
dvr=zeros(2,1);
%DEFORMATION INCREMENTS OR DEFORMATION RATES
      dvax=cosa*(ddise(4,1)-ddise(1,1))+sina*(ddise(5,1)-ddise(2,1));
      rot=(sina*(ddise(4,1)-ddise(1,1))+cosa*(ddise(2,1)-ddise(5,1)))/f1;
      dvr(1,1)=ddise(3,1)+rot;
      dvr(2,1)=ddise(6,1)+rot;
%%

== matlab function Generate Element Restoring Forces/Generate Type 4 Element Restoring Force Element 7/Type 4 Element RF ==
  data: TotalRF output inherited; Element input inherited; NumFreeDOF parameter inherited; Displacement input inherited
% get restoring force for the element
% returns (6x1) restoring force vector of element in global coordinates
function TotalRF  = eml(Element, NumFreeDOF, Displacement)

%% Input mapping
K11 = Element(1);
K12 = Element(2);
K21 = Element(3);
K22 = Element(4);
Node1UX = Element(5);
Node1UY = Element(6);
Node1THETA = Element(7);
Node2UX = Element(8);
Node2UY = Element(9);
Node2THETA = Element(10);

% preset arrays
SE = zeros(6,6);
    
SE(1, 1) = K11;
SE(1, 4) = K12;
SE(4, 1) = K21;
SE(4, 4) = K22;

%create the displacement Ue (6x1) vector of the element in global coordinates
Ue = zeros(6, 1);
dof=zeros(6,1);
dof(1,1)=Node1UX;
dof(2,1)=Node1UY;
dof(3,1)=Node1THETA;
dof(4,1)=Node2UX;
dof(5,1)=Node2UY;
dof(6,1)=Node2THETA;
for i=1:6
    if dof(i,1)<=NumFreeDOF
        Ue(i,1)=Displacement(dof(i,1),1);
    end
end
RF = SE * Ue;  %resisting (6x1) resisting force vector of element in global coordinates

% Form total restoring force vector
TotalRF = zeros(NumFreeDOF, 1);
    
% Get element nodes to assemble in the structure restoring force vector
if Node1UX <= NumFreeDOF
    TotalRF(Node1UX, 1) = RF(1, 1);
end
if Node1UY <= NumFreeDOF
    TotalRF(Node1UY, 1) = RF(2, 1);
end
if Node1THETA <= NumFreeDOF
    TotalRF(Node1THETA, 1) = RF(3, 1);
end
if Node2UX <= NumFreeDOF
    TotalRF(Node2UX, 1) = RF(4, 1);
end
if Node2UY <= NumFreeDOF
    TotalRF(Node2UY, 1) = RF(5, 1);
end
if Node2THETA <= NumFreeDOF
    TotalRF(Node2THETA, 1) = RF(6, 1);
end
